simulink model "sgMdl_IO134_AnalogInputsDigitalLoopback"  (R2024b)
settings: Solver=FixedStepAuto  StartTime=0.0  StopTime=inf  RelTol=1e-3  EnableMultiTasking=on
libraries: speedgoatlib_IO134 x4
Description:
  | IO134 - Analog Inputs and Digital Loopback
settings Model: sg_rtwmakecfg_data=_sglibc_  ModifiedByFormat=Speedgoat  Creator=Speedgoat  LastModifiedBy=Speedgoat
settings SolverCC: ConcurrentTasks=on  AlgebraicLoopSolver=TrustRegion  PositivePriorityOrder=on  AutoInsertRateTranBlk=on  InsertRTBMode=Never (minimum delay)
settings DataIOCC: SaveFormat=StructureWithTime  ReturnWorkspaceOutputs=off
settings OptimizationCC: BlockReduction=off  OptimizeBlockIOStorage=off  BufferReuse=off  ReuseModelBlockBuffer=off  GlobalBufferReuse=off  ExpressionFolding=off  LocalBlockOutputs=off
settings DebuggingCC: TasksWithSamePriorityMsg=none  UnconnectedInputMsg=warning  UnconnectedOutputMsg=warning  UnconnectedLineMsg=warning  ArithmeticOperatorsInVariantConditions=warning
settings HardwareCC: ProdBitPerLong=64  ProdLongLongMode=on  ProdHWDeviceType=Intel->x86-64 (Linux 64)
settings ModelReferenceCC: EnableRefExpFcnMdlSchedulingChecks=on
settings SFSimCC: SimUseLocalCustomCode=off  CustomCodeUndefinedFunction=UseInterfaceOnly
settings RTWCC: Description=Speedgoat Real-Time Target Machine  SystemTargetFile=speedgoat.tlc  TemplateMakefile=slrealtime_default_tmf  RTWUseLocalCustomCode=off  Toolchain=Simulink Real-Time Toolchain  BuildConfiguration=Faster Runs  TargetLang=C++  GPUComputeCapability=3.5  DLArmComputeVersion=19.05
settings CodeAppCC: StateflowObjectComments=on
settings SimulinkRealTimeTargetCC: SubcomponentCodeInterfacePackaging=Reusable function  InstructionSetFMA=off  LogToMDFFile=off  SLRTFileLogMaxRuns=10  UseGCCFastMath=on
settings ConfigComp: CovBoundaryAbsTol=1.0e-5

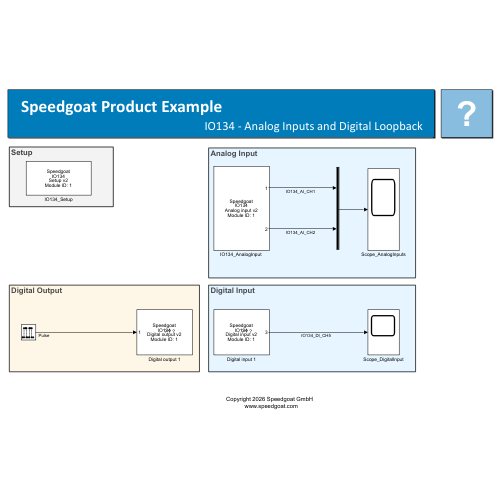
[thumbnail: Simulink's stored preview of the top-level diagram]
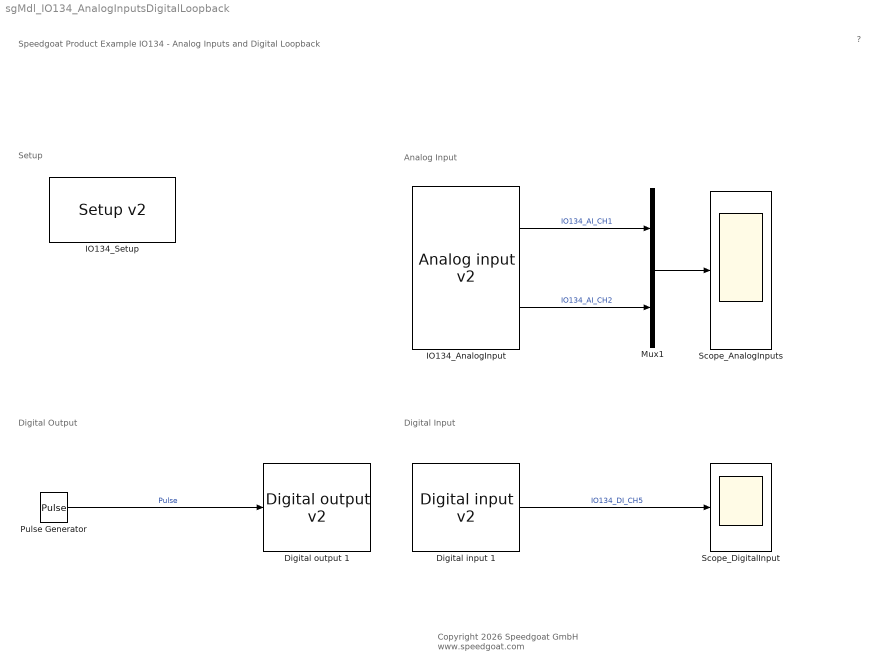
== system sgMdl_IO134_AnalogInputsDigitalLoopback ==
  note: Setup
  note: Analog Input
  note: Digital Output
  note: Digital Input
  note: Speedgoat Product Example
      | IO134 - Analog Inputs and Digital Loopback
  note: ?
  note: Copyright 2026 Speedgoat GmbH
      |  www.speedgoat.com
  Digital input 1 : speedgoatlib_IO134/Digital input v2   parModuleId=1  parSampleTime=0.001  parPciSlot=-1  parDiChannels=5
      settings: SourceProductName=Simulink Real-Time: Speedgoat I/O Blockset
  Digital output 1 : speedgoatlib_IO134/Digital output v2   parModuleId=1  parSampleTime=0.001  parPciSlot=-1  parDoChannels=1  parDoInitValues=0  parDoReset=1
      settings: SourceProductName=Simulink Real-Time: Speedgoat I/O Blockset
  "IO134_AnalogInput " : speedgoatlib_IO134/Analog input v2   parModuleId=1  parSampleTime=0.001  parPciSlot=-1  parAdcChannels=[1 2]  parAdcVoltageRange=[2 2 2 2]  parAdcOversamplRate=[1 1 1 1]  parAdcContSampling=0  parAdcDmaEnable=0  parAdcActiveDmaDevices=[1 1 1 1]  parAdcFrameSize=100
      settings: SourceProductName=Simulink Real-Time: Speedgoat I/O Blockset
  IO134_Setup : speedgoatlib_IO134/Setup v2   parPciSlot=-1  parModuleId=1  parInterModuleSync=None  parConvClockBaseRate=20MHz  parConvClock1Divider=20000  parConvClock2Divider=20000  parFrameTriggerEnable=off  parFrameTriggerDivider=10  parConvClock1BaseRate=1  parConvClock2BaseRate=1  parFrameTriggerClock=1  parAdcChannels=[1 2]  parAdcRange1=+-10V  parAdcRange2=+-10V  parAdcRange3=+-10V  parAdcRange4=+-10V  parAdcVoltageRange=[2 2 2 2]  parAdcOversampling1=None  parAdcOversampling2=None  parAdcOversampling3=None  parAdcOversampling4=None  parAdcOversamplRate=[1 1 1 1]  parAdcContSampling=off  parAdcDataCorrection=Automatic  parAdcCorrectionActive={}  parAdcCorrectionPm5V={'1','0','0';'2','0','0';'3','0','0';'4','0','0';'5','0','0';'6','0','0';'7','0','0';'8','0','0';'9','0','0';'10','0','0';'11','0','0';'12','0','0';'13','0','0';'14','0','0';'15','0','0';'16','0','0';'17','0','0';'18','0','0';'19','0','0';'20','0','0';'21','0','0';'22','0','0';'23','0','0';'24','0','0';'25','0','0';'26','0','0';'27','0','0';'28','0','0';'29','0','0';'30','0','0';'31','0','0';'32','0','0'}  parAdcCorrectionPm10V={'1','0','0';'2','0','0';'3','0','0';'4','0','0';'5','0','0';'6','0','0';'7','0','0';'8','0','0';'9','0','0';'10','0','0';'11','0','0';'12','0','0';'13','0','0';'14','0','0';'15','0','0';'16','0','0';'17','0','0';'18','0','0';'19','0','0';'20','0','0';'21','0','0';'22','0','0';'23','0','0';'24','0','0';'25','0','0';'26','0','0';'27','0','0';'28','0','0';'29','0','0';'30','0','0';'31','0','0';'32','0','0'}  parAdcDmaEnable=off  parAdcDmaClock=Clock 1  parAdcFrameSize_=100  parAdcSampleTime_=-1  parAdcActiveDmaDevices=[1 1 1 1]  parAdcFrameTriggerEnable=0  parAdcFrameSize=100  parAdcSampleTime=0.1  parDacChannels=[]  parDacInitValues=0  parDacReset=0  parDacVoltageRange=zeros(1,0)  parDacSyncOut=on  parDacDataCorrection=Automatic  parDacDmaEnable=off  parDacDmaLatency=Until next frame  parDacDmaClock=Clock 1  parDacFrameSize_=100  parDacSampleTime_=-1  parDacActiveDmaDevices=[]  parDacFrameTriggerEnable=0  parDacFrameSize=100  parDacSampleTime=0.1  parDoChannels=[1]  parDoInitValues=0  parDoReset=1  parDiChannels=[5]  parDiDebounceEnable=off  parDiDebounceTime=0  parDiDebounceValue=0  parDioPullRefFront=Pull-up 3.3V  parDioPullRefRear=Floating
      settings: SourceProductName=Simulink Real-Time: Speedgoat I/O Blockset
  Mux1 : Mux  Inputs=2
  Pulse Generator : DiscretePulseGenerator  Period=10  PulseWidth=5  SampleTime=0.001
  Scope_AnalogInputs : Scope
  Scope_DigitalInput : Scope
  wires:
  Mux1/1 -> Scope_AnalogInputs/1
  "IO134_AnalogInput "/2 -> Mux1/2  "IO134_AI_CH2"
  Pulse Generator/1 -> Digital output 1/1  "Pulse"
  "IO134_AnalogInput "/1 -> Mux1/1  "IO134_AI_CH1"
  Digital input 1/1 -> Scope_DigitalInput/1  "IO134_DI_CH5"
